simulink model "throttle_real_1"  (Simulink 8.3)
settings: Solver=ode4  StartTime=0.0  StopTime=2  FixedStep=0.002  RelTol=1e-3
undefined symbols (not defined in the file or in its folder): DiscIntNeverNeededParam, mpccontroller
libraries: simulink x2
settings Model: Creator=jinwei_copy  LastModifiedBy=Administrator  BufferReuse=off
settings SolverCC: AlgebraicLoopSolver=LineSearch
settings OptimizationCC: BlockReduction=off  BooleanDataType=off  ConditionallyExecuteInputs=off  OptimizeBlockIOStorage=off  BufferReuse=off  GlobalBufferReuse=off  ExpressionFolding=off  ExpressionDepthLimit=2147483647  LocalBlockOutputs=off
settings DebuggingCC: FcnCallInpInsideContextMsg=UseLocalSettings
settings SFSimCC: SimParseCustomCode=off

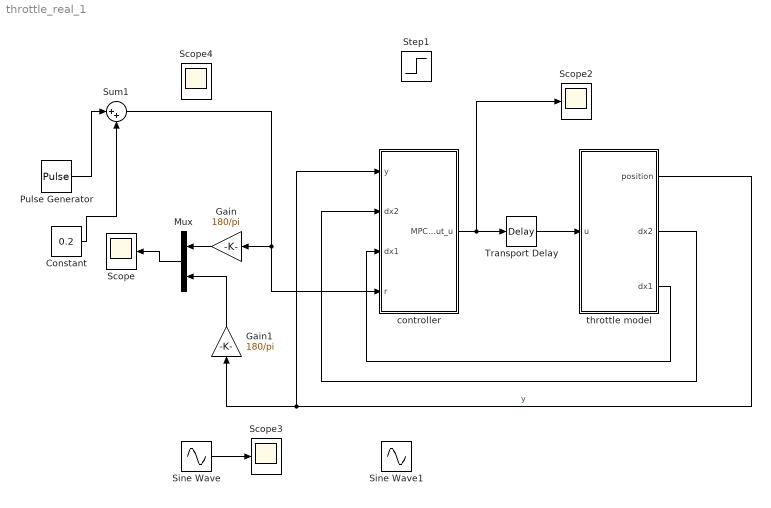
== system throttle_real_1 ==
  Constant : Constant  Value=0.2
  Gain : Gain  Gain=180/pi
  Gain1 : Gain  Gain=180/pi
  Mux : Mux  Inputs=2
  Pulse Generator : DiscretePulseGenerator  Amplitude=1.2  Period=800  PulseWidth=400  SampleTime=0.002
  Scope{,2..4} (4 alike) : Scope
      Scope settings: TimeRange=2  YMin=80.185  YMax=80.2325  SaveName=EXP  SampleInput=on
      Scope2 settings: TimeRange=2  YMin=0.595  YMax=0.635  SaveName=EXP2  SampleInput=on
      Scope3 settings: TimeRange=1  YMin=-0.25  SaveName=EXP3  SampleInput=on
      Scope4 settings: TimeRange=1  YMin=0.1  YMax=1.1  SaveName=EXP5  SampleInput=on
  Sine Wave : Sin  Amplitude=0.5  Bias=0.5  Frequency=10  SampleTime=0
  Sine Wave1 : Sin  Amplitude=0.5  Bias=0.5  Frequency=10  SampleTime=0
  Step1 : Step  Time=0.3  Before=0.1  SampleTime=0
  Sum1 : Sum  Inputs=|++
  Transport Delay : TransportDelay  DelayTime=0
  controller : Subsystem
      mask init:
      | % n=16.95;
      | % kt=0.0183;
      | % kv=kt;
      | % kf=0.2999*kt;
      | % kpre=0.3942*kt*n;
      | % ks=0.0011*kt*n;
      | % J=(4.0e-5)*pi/180;
      | % B=(2.4e-4)*pi/180;
      | % 
      | % k1=200;
      | % k2=200;
  throttle model : Subsystem  TreatAsAtomicUnit=on
      mask init:
      | switch 'a'          %input gear here
      | 	case 'a'
      | 		n=22.08;
      | 		%c=63.662;
      |         c=1;
      | 		Vbat=12;
      | 		kt=0.0183;
      | 		kv=kt;
      | 		kf=0.2999*kt;
      | 		kpre=0.3942*kt*n;
      | 		ksa=0.0011*kt*n*c;
      | 		ksb=0.0093*kt*n*c;
      | 		J=4e-6;
      | 		B=2.4e-5;
      | 		defult=0.108;
      | 	case 'b'
      | 		n=22.08;
      | 		kt=0.0183;
      | 		kv=kt;
      | 		kf=0.2999*kt;
      | 		kpre=0.3942*kt*n;
      | 		ks=0.0093*kt*n;
      | 		J=4.0e-5;
      | 		B=2.4e-4;
      | 		defult=0.116;
      | 	otherwise
      | 		disp('gear error.')
      | end
  wires:
  throttle model/1(position) -> Gain1/1, controller/1(y)  "y"
  throttle model/2(dx2) -> controller/2(dx2)
  throttle model/3(dx1) -> controller/3(dx1)
  Mux/1 -> Scope/1
  Constant/1 -> Sum1/2
  Pulse Generator/1 -> Sum1/1
  Sine Wave/1 -> Scope3/1
  Gain/1 -> Mux/1
  Gain1/1 -> Mux/2
  Sum1/1 -> controller/4(r), Gain/1
  controller/1(MPC_Out_u) -> Transport Delay/1, Scope2/1
  Transport Delay/1 -> throttle model/1(u)

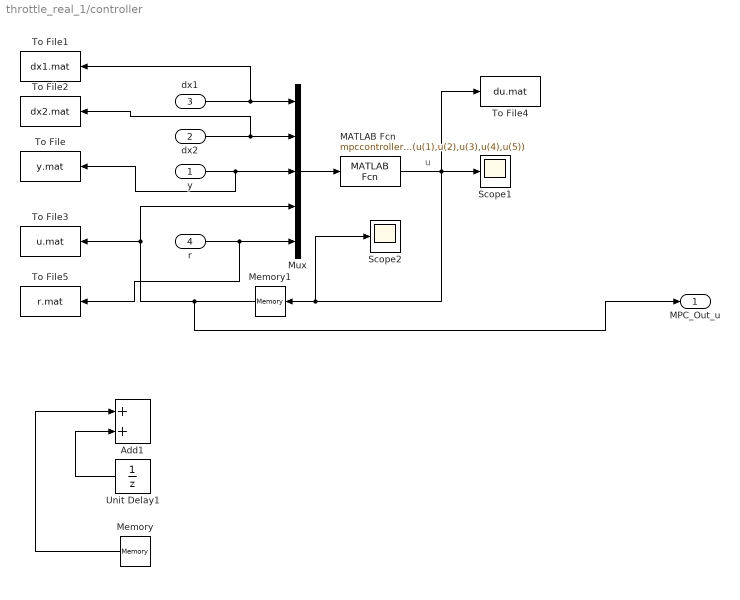
== system throttle_real_1/controller ==
  note: u
  y : Inport
  dx2 : Inport  Port=2
  dx1 : Inport  Port=3
  r : Inport  Port=4
  Add1 : Sum
  MATLAB Fcn : MATLABFcn  MATLABFcn=mpccontroller(u(1),u(2),u(3),u(4),u(5))
  Memory : Memory  InheritSampleTime=on
  Memory1 : Memory  InheritSampleTime=on  LinearizeMemory=on  LinearizeAsDelay=on
  Mux : Mux  Inputs=5
  Scope1 : Scope
      settings: YMin=-3e-05  YMax=4.5e-05  SaveName=du
  Scope2 : Scope
      settings: TimeRange=0.1361256544502618  YMin=0.1540901502504175  YMax=0.5794657762938231
  To File : ToFile  Filename=y.mat  MatrixName=y
  To File1 : ToFile  Filename=dx1.mat  MatrixName=dx1
  To File2 : ToFile  Filename=dx2.mat  MatrixName=dx2
  To File3 : ToFile  Filename=u.mat  MatrixName=u
  To File4 : ToFile  Filename=du.mat  MatrixName=du
  To File5 : ToFile  Filename=r.mat  MatrixName=r
  Unit Delay1 : UnitDelay  SampleTime=-1
  MPC_Out_u : Outport
  wires:
  dx1/1 -> Mux/1, To File1/1
  y/1 -> Mux/3, To File/1
  MATLAB Fcn/1 -> Memory1/1, Scope2/1, To File4/1, Scope1/1
  dx2/1 -> Mux/2, To File2/1
  Mux/1 -> MATLAB Fcn/1
  r/1 -> To File5/1, Mux/5
  Unit Delay1/1 -> Add1/2
  Memory/1 -> Add1/1
  Memory1/1 -> MPC_Out_u/1, Mux/4, To File3/1

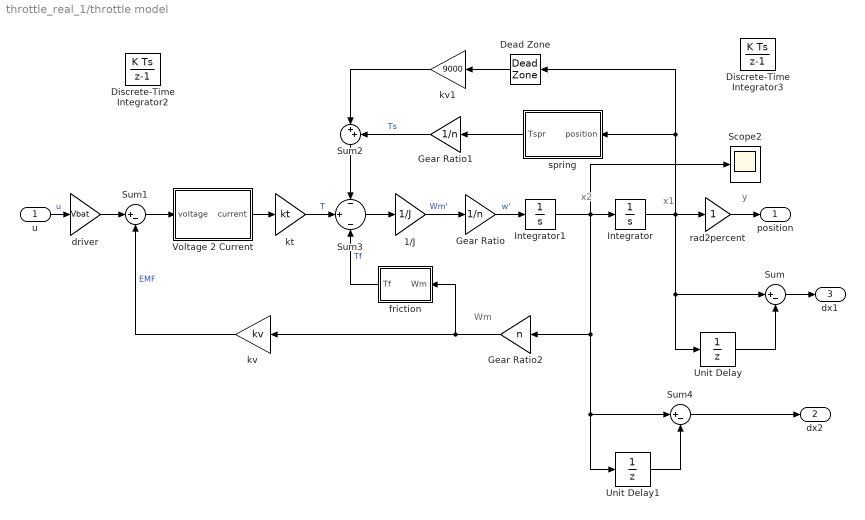
== system throttle_real_1/throttle model ==
  note: x2
  note: x1
  note: y
  note: Wm
  u : Inport
  1/J : Gain  Gain=1/J
  Dead Zone : DeadZone  LowerValue=0  UpperValue=100/c  SaturateOnIntegerOverflow=on
  Discrete-Time Integrator2 : DiscreteIntegrator  SampleTime=-1  ICPrevOutput=DiscIntNeverNeededParam  ICPrevScaledInput=DiscIntNeverNeededParam
  Discrete-Time Integrator3 : DiscreteIntegrator  InitialCondition=defult  SampleTime=-1  ICPrevOutput=DiscIntNeverNeededParam  ICPrevScaledInput=DiscIntNeverNeededParam
  Gear Ratio : Gain  Gain=1/n  SaturateOnIntegerOverflow=on  OutDataTypeStr=Inherit: Same as input  ParamDataTypeStr=Inherit: Same as input
  Gear Ratio1 : Gain  Gain=1/n  SaturateOnIntegerOverflow=on  OutDataTypeStr=Inherit: Same as input  ParamDataTypeStr=Inherit: Same as input
  Gear Ratio2 : Gain  Gain=n  SaturateOnIntegerOverflow=on  OutDataTypeStr=Inherit: Same as input  ParamDataTypeStr=Inherit: Same as input
  Integrator : Integrator
  Integrator1 : Integrator
  Scope2 : Scope
      settings: TimeRange=1  YMin=-0.25  SaveName=EXP4  SampleInput=on
  Sum : Sum  Inputs=|+-
  Sum1 : Sum  Inputs=|+-  SaturateOnIntegerOverflow=on  InputSameDT=on  OutDataTypeStr=Inherit: Same as first input
  Sum2 : Sum  Inputs=|++  SaturateOnIntegerOverflow=on  InputSameDT=on  OutDataTypeStr=Inherit: Same as first input
  Sum3 : Sum  Inputs=-|+|-  SaturateOnIntegerOverflow=on  InputSameDT=on  OutDataTypeStr=Inherit: Same as first input
  Sum4 : Sum  Inputs=|+-
  Unit Delay : UnitDelay  SampleTime=-1
  Unit Delay1 : UnitDelay  SampleTime=-1
  Voltage 2 Current : Subsystem
  driver : Gain  Gain=Vbat
  friction : Subsystem
  kt : Gain  Gain=kt  SaturateOnIntegerOverflow=on  OutDataTypeStr=Inherit: Same as input  ParamDataTypeStr=Inherit: Same as input
  kv : Gain  Gain=kv  SaturateOnIntegerOverflow=on  OutDataTypeStr=Inherit: Same as input  ParamDataTypeStr=Inherit: Same as input
  kv1 : Gain  Gain=9000  SaturateOnIntegerOverflow=on  OutDataTypeStr=Inherit: Same as input  ParamDataTypeStr=Inherit: Same as input
  rad2percent : Gain  SaturateOnIntegerOverflow=on  OutDataTypeStr=Inherit: Same as input  ParamDataTypeStr=Inherit: Same as input
  spring : Subsystem
  position : Outport  InitialOutput=defult
  dx2 : Outport  Port=2  InitialOutput=defult
  dx1 : Outport  Port=3  InitialOutput=defult
  wires:
  u/1 -> driver/1  "u"
  driver/1 -> Sum1/1
  Sum1/1 -> Voltage 2 Current/1(voltage)
  Voltage 2 Current/1(current) -> kt/1
  kt/1 -> Sum3/2  "T"
  Sum3/1 -> 1/J/1
  1/J/1 -> Gear Ratio/1  "Wm'"
  Gear Ratio/1 -> Integrator1/1  "w'"
  Integrator1/1 -> Integrator/1, Gear Ratio2/1, Sum4/1, Unit Delay1/1, Scope2/1
  Integrator/1 -> rad2percent/1, spring/1(position), Dead Zone/1, Sum/1, Unit Delay/1
  spring/1(Tspr) -> Gear Ratio1/1
  rad2percent/1 -> position/1
  friction/1(Tf) -> Sum3/3  "Tf"
  kv/1 -> Sum1/2  "EMF"
  Gear Ratio1/1 -> Sum2/2  "Ts"
  Gear Ratio2/1 -> friction/1(Wm), kv/1
  Dead Zone/1 -> kv1/1
  Sum2/1 -> Sum3/1
  kv1/1 -> Sum2/1
  Unit Delay/1 -> Sum/2
  Sum/1 -> dx1/1
  Unit Delay1/1 -> Sum4/2
  Sum4/1 -> dx2/1

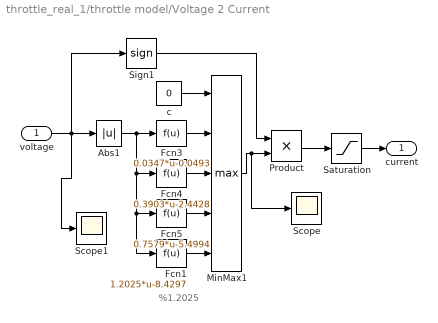
== system throttle_real_1/throttle model/Voltage 2 Current ==
  note: %1.2025
  voltage : Inport
  Abs1 : Abs
  Fcn1 : Fcn  Expr=1.2025*u-8.4297
  Fcn3 : Fcn  Expr=0.0347*u-0.0493
  Fcn4 : Fcn  Expr=0.3903*u-2.4428
  Fcn5 : Fcn  Expr=0.7579*u-5.4994
  MinMax1 : MinMax  Function=max  Inputs=5
  Product : Product  RndMeth=Zero
  Saturation : Saturate  UpperLimit=6  LowerLimit=-6
  Scope : Scope
      settings: SaveName=ScopeData2
  Scope1 : Scope
      settings: SaveName=ScopeData3
  Sign1 : Signum  ZeroCross=off
  c : Constant  Value=0
  current : Outport
  wires:
  voltage/1 -> Sign1/1, Abs1/1, Scope1/1
  Fcn5/1 -> MinMax1/4
  Abs1/1 -> Fcn3/1, Fcn4/1, Fcn5/1, Fcn1/1
  Sign1/1 -> Product/1
  MinMax1/1 -> Product/2, Scope/1
  Fcn4/1 -> MinMax1/3
  Fcn3/1 -> MinMax1/2
  c/1 -> MinMax1/1
  Product/1 -> Saturation/1
  Fcn1/1 -> MinMax1/5
  Saturation/1 -> current/1

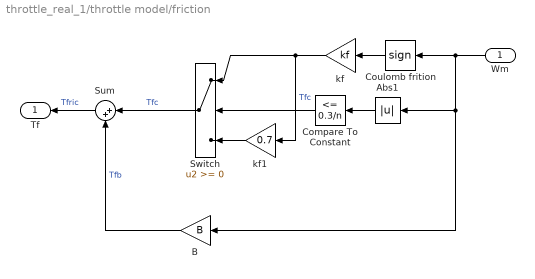
== system throttle_real_1/throttle model/friction ==
  Wm : Inport
  Abs1 : Abs
  B : Gain  Gain=B  SaturateOnIntegerOverflow=on  OutDataTypeStr=Inherit: Same as input  ParamDataTypeStr=Inherit: Same as input
  Compare To Constant : simulink/Logic and Bit Operations/Compare To Constant  relop=<=  const=0.3/n  OutDataTypeStr=uint8  ZeroCross=off
  Coulomb frition : Signum  ZeroCross=off
  Sum : Sum  Inputs=|++  SaturateOnIntegerOverflow=on  InputSameDT=on  OutDataTypeStr=Inherit: Same as first input
  Switch : Switch
  kf : Gain  Gain=kf  SaturateOnIntegerOverflow=on  OutDataTypeStr=Inherit: Same as input  ParamDataTypeStr=Inherit: Same as input
  kf1 : Gain  Gain=0.7  SaturateOnIntegerOverflow=on  OutDataTypeStr=Inherit: Same as input  ParamDataTypeStr=Inherit: Same as input
  Tf : Outport
  wires:
  Coulomb frition/1 -> kf/1
  Wm/1 -> Coulomb frition/1, B/1, Abs1/1
  Switch/1 -> Sum/1  "Tfc"
  B/1 -> Sum/2  "Tfb"
  Sum/1 -> Tf/1  "Tfric"
  Abs1/1 -> Compare To Constant/1
  Compare To Constant/1 -> Switch/2
  kf/1 -> Switch/1, kf1/1  "Tfc"
  kf1/1 -> Switch/3

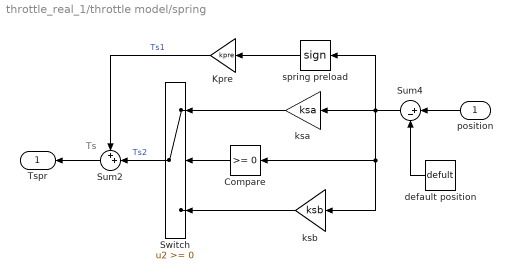
== system throttle_real_1/throttle model/spring ==
  note: Ts
  position : Inport
  Compare : simulink/Logic and Bit Operations/Compare To Zero  relop=>=  OutDataTypeStr=uint8  ZeroCross=off
  Kpre : Gain  Gain=kpre  SaturateOnIntegerOverflow=on  OutDataTypeStr=Inherit: Same as input  ParamDataTypeStr=Inherit: Same as input
  Sum2 : Sum  Inputs=++|  SaturateOnIntegerOverflow=on  InputSameDT=on  OutDataTypeStr=Inherit: Same as first input
  Sum4 : Sum  Inputs=|+-  SaturateOnIntegerOverflow=on  InputSameDT=on  OutDataTypeStr=Inherit: Same as first input
  Switch : Switch
  default position : Constant  Value=defult  SampleTime=-1
  ksa : Gain  Gain=ksa  SaturateOnIntegerOverflow=on  OutDataTypeStr=Inherit: Same as input  ParamDataTypeStr=Inherit: Same as input
  ksb : Gain  Gain=ksb  SaturateOnIntegerOverflow=on  OutDataTypeStr=Inherit: Same as input  ParamDataTypeStr=Inherit: Same as input
  spring preload : Signum  ZeroCross=off
  Tspr : Outport
  wires:
  spring preload/1 -> Kpre/1
  ksa/1 -> Switch/1
  ksb/1 -> Switch/3
  Compare/1 -> Switch/2
  Switch/1 -> Sum2/2  "Ts2"
  Kpre/1 -> Sum2/1  "Ts1"
  Sum2/1 -> Tspr/1
  position/1 -> Sum4/1
  default position/1 -> Sum4/2
  Sum4/1 -> ksa/1, spring preload/1, ksb/1, Compare/1
